simulink model "f2837x_cmpss"  (R2021b)
settings: Solver=FixedStepDiscrete  StartTime=0.0  StopTime=Inf  RelTol=1e-3  EnableMultiTasking=on
libraries: c2837xDlib x4, simulink x2, demo_controls x1
settings Model: ExtModeTrigDuration=8  Creator=The MathWorks, Inc.  LastModifiedBy=The MathWorks, Inc.
settings SolverCC: AlgebraicLoopSolver=TrustRegion
settings OptimizationCC: DefaultUnderspecifiedDataType=single  EnhancedBackFolding=on  PassReuseOutputArgsAs=Individual arguments  MaxStackSize=1024  OptimizeBlockOrder=speed  DifferentSizesBufferReuse=on  OptimizationCustomize=off  DenormalBehavior=FlushToZero  EfficientTunableParamExpr=on
settings DebuggingCC: ParameterTunabilityLossMsg=error  SFMachineParentedDataDiag=warning
settings HardwareCC: ProdBitPerChar=16  ProdBitPerInt=16  ProdBitPerPointer=32  ProdBitPerSizeT=32  ProdBitPerPtrDiffT=32  ProdLargestAtomicInteger=Integer  ProdLargestAtomicFloat=None  ProdWordSize=16  ProdLongLongMode=on  ProdHWDeviceType=Texas Instruments->C2000
settings SFSimCC: MATLABDynamicMemAlloc=off
settings RTWCC: Description=Embedded Coder  SystemTargetFile=ert.tlc  HardwareBoard=TI Delfino F28379D LaunchPad  TemplateMakefile=ert_default_tmf  Toolchain=Texas Instruments Code Composer Studio (C2000)
settings CodeAppCC: ForceParamTrailComments=on  IgnoreCustomStorageClasses=off  OperatorAnnotations=on  SimulinkDataObjDesc=on  SFDataObjDesc=on  InsertBlockDesc=on
settings ERTTargetCC: CodeReplacementLibrary=TI C28x  ExtModeTransport=4  ExtModeStaticAlloc=on  ExtModeStaticAllocSize=10000  ExtModeMexFile=ext_xcp  ExtModeIntrfLevel=Level2 - Open

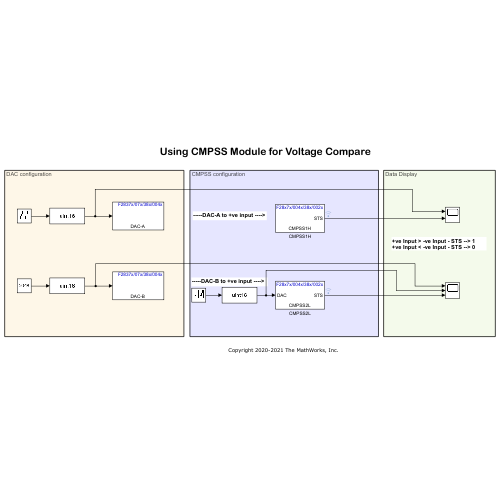
[thumbnail: Simulink's stored preview of the top-level diagram]
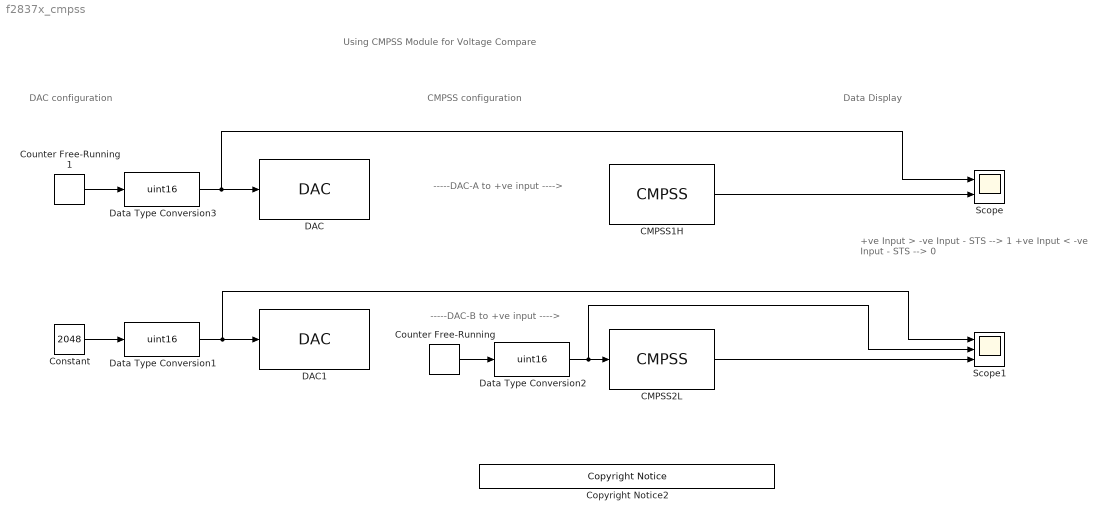
== system f2837x_cmpss ==
  note: +ve Input > -ve Input - STS --> 1
      | +ve Input < -ve Input - STS --> 0
  note: DAC configuration
  note: Data Display
  note: CMPSS configuration
  note: Using CMPSS Module for Voltage Compare
  note: -----DAC-A to +ve input ---->
  note: -----DAC-B to +ve input ---->
  CMPSS1H : c2837xDlib/CMPSS  Priority=3  Module=CMPSS1_COMPH  NegativeInput=Internal DAC  DacValueSourceSel=DAC module  DacValueVia=Dialog  DACHValue=2048  DACLValue=0  RampMaxRefVal=0  RampDecVal=0  RampDelayVal=0  EnableLatchOut=off  EnableLatchClear=off  SampleTime=-1
      settings: SourceProductBaseCode=TIC2000
  CMPSS2L : c2837xDlib/CMPSS  Priority=3  Module=CMPSS2_COMPL  NegativeInput=Internal DAC  DacValueSourceSel=DAC module  DacValueVia=Input port  DACHValue=2048  DACLValue=0  RampMaxRefVal=0  RampDecVal=0  RampDelayVal=0  EnableLatchOut=off  EnableLatchClear=off  SampleTime=-1
      settings: SourceProductBaseCode=TIC2000
  Constant : Constant  Value=2048
  Copyright Notice2 : demo_controls/Copyright Notice  year=2020  prod=tic2000
      settings: SourceProductBaseCode=ME
  Counter Free-Running : simulink/Sources/Counter Free-Running  NumBits=12  tsamp=0.01
  Counter Free-Running1 : simulink/Sources/Counter Free-Running  NumBits=12  tsamp=-1
  DAC : c2837xDlib/DAC  Priority=1  channel=A  saturate=off
      settings: SourceProductBaseCode=TIC2000
  DAC1 : c2837xDlib/DAC  Priority=1  channel=B  saturate=off
      settings: SourceProductBaseCode=TIC2000
  Data Type Conversion1 : DataTypeConversion  OutDataTypeStr=uint16
  Data Type Conversion2 : DataTypeConversion  OutDataTypeStr=uint16
  Data Type Conversion3 : DataTypeConversion  OutDataTypeStr=uint16
  Scope : Scope  NumInputPorts=2
  Scope1 : Scope  NumInputPorts=3
  wires:
  CMPSS1H/1 -> Scope/2
  Data Type Conversion1/1 -> DAC1/1, Scope1/1
  Constant/1 -> Data Type Conversion1/1
  Counter Free-Running/1 -> Data Type Conversion2/1
  Data Type Conversion2/1 -> CMPSS2L/1, Scope1/2
  Data Type Conversion3/1 -> DAC/1, Scope/1
  CMPSS2L/1 -> Scope1/3
  Counter Free-Running1/1 -> Data Type Conversion3/1
